simulink model "sim1"  (Simulink 6.0)
settings: Solver=ode45  StartTime=0.0  StopTime=30  RelTol=1e-3
settings Model: LastModifiedBy=aluno

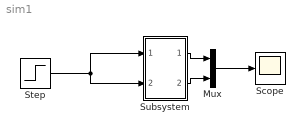
== system sim1 ==
  Mux : Mux  Inputs=2
  Scope : Scope
  Step : Step  Time=0  SampleTime=0
  Subsystem : Subsystem  mask{K=0, R1=50*(10^3), R2=50*(10^3), C1=250*(10^-9), C2=250*(10^-9)}
      mask prompts: K "K=R4/R3"; R1 "Resistencia R1"; R2 "Resistencia R2"; C1 "Capacitor C1"; C2 "Capacitor C2"
  wires:
  Step/1 -> Subsystem/1(In1), Subsystem/2(In2)
  Subsystem/1(Out1) -> Mux/1
  Subsystem/2(Out2) -> Mux/2
  Mux/1 -> Scope/1

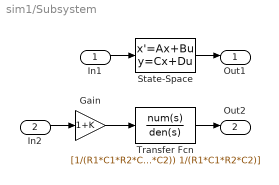
== system sim1/Subsystem ==
  In1 : Inport  Port=1  LatchInput=off
  In2 : Inport  Port=2  LatchInput=off
  Gain : Gain  Gain=1+K
  State-Space : StateSpace  A=[ ((-1/R1*C1)-(1/R2*C1)) ((1+K)*(1/(R1*C1))+((K)*(1/(R2*C1)))); -1/(R2*C2) (K)*(1/(R2*C2)) ]  B=[-1/(R1*C1); 0]  C=[0 (1+K)]  D=0
  Transfer Fcn : TransferFcn  Numerator=[1/(R1*C1*R2*C2)]  Denominator=[1 (1/(R1*C1)+1/(R2*C1)-(K)*1/(R2*C2)) 1/(R1*C1*R2*C2)]
  Out1 : Outport
  Out2 : Outport  Port=2
  wires:
  Gain/1 -> Transfer Fcn/1
  In1/1 -> State-Space/1
  State-Space/1 -> Out1/1
  In2/1 -> Gain/1
  Transfer Fcn/1 -> Out2/1
